simulink model "Doppelpendel_EKF"  (R2020b)
settings: Solver=ode45  StartTime=0.0  StopTime=10  EnableMultiTasking=on
undefined symbols (not defined in the file or in its folder): parDP, parEKF, parLQR
libraries: cstblocks x3
(part 2 of 2)

== matlab function Doppelpendel_EKF/Regler/LQR+EKF ==
  settings: updateMethod=DISCRETE  sampleTime=parLQR.Ta
  data: Switch_Rueckfuehrung input; statesd input; states input; uFF input; uG output; parDP parameter; parLQR parameter; parEKF parameter; xestout output; e_phi1 output; e_s output; e output; Pplus output
function [uG,xestout,e_phi1,e_s,e,Pplus]  = LQG(Switch_Rueckfuehrung,statesd,states,uFF,parDP,parLQR,parEKF)

%Anfangsbedinungen = Ruhelagen
persistent xI
if isempty(xI) xI = double(0); end

persistent xminus
if isempty(xminus)xminus = [parEKF.phi10;parEKF.omega10;parEKF.phi20;parEKF.omega20;parEKF.s0;parEKF.w0]; end

persistent Pminus
if isempty( Pminus) Pminus = diag([parEKF.delta,parEKF.delta,parEKF.delta,parEKF.delta,parEKF.delta,parEKF.delta]); end

%Ausgang
xestout=xminus;

%%%%%%%%%%%%%%%%%%%%%%%%%%%%%%%%%%%%%%%%%%%%%%%%%%%%%%%%%%%%%%%%%%%%%%%%%%%
%LQR-Regler
%%%%%%%%%%%%%%%%%%%%%%%%%%%%%%%%%%%%%%%%%%%%%%%%%%%%%%%%%%%%%%%%%%%%%%%%%%%

% Folgendes hier bitte ausführen:
% 1.) PI-Zustandsregler einfügen
    xI = xI + (statesd(5) - xestout(5));
    %Gesamtrückführung
    uFB = parLQR.kx*(xestout - statesd) + parLQR.kI * xI;
    uG = uFB + uFF;  

%%%%%%%%%%%%%%%%%%%%%%%%%%%%%%%%%%%%%%%%%%%%%%%%%%%%%%%%%%%%%%%%%%%%%%%%%%%
%EKF
%%%%%%%%%%%%%%%%%%%%%%%%%%%%%%%%%%%%%%%%%%%%%%%%%%%%%%%%%%%%%%%%%%%%%%%%%%%

% Folgendes hier bitte ausführen:
% 1.) Extended-Kalman-Filter einfügen
    C_k = [1 0 0 0 0 0; 0 0 0 0 1 0];
    % Hk = 0;
    %Korrekturschritt
    L_k = Pminus*C_k' / (C_k*Pminus*C_k' + parEKF.Rn);
    xplus = xminus + L_k*( [states(1); states(5)] - [ xestout(1); xestout(5)] );
    Pplus = (eye(6) - L_k*C_k) * Pminus;

    %Prädiktorschritt
    Phi_k = eye(6) + parDP.Ta*fcnAsys(xplus,uG,parDP);
    xminus = xplus + parDP.Ta*fcnfx(xplus,uG,parDP);
    Pminus = Phi_k*Pplus*Phi_k' + parEKF.Qn;


    e_phi1 = states(1) - xminus(1);
    e_s = states(5)- xminus(5);
    e = [e_phi1 ;0; 0; 0; e_s ;0];

end

%% Rechte Seite
function fx = fcnfx(xplus,uG,parDP)

    InvD11 = parDP.m2*parDP.a2*parDP.a2+parDP.J2;
    InvD12 = -parDP.m2*parDP.l1*parDP.a2*cos(xplus(1)-xplus(3));
    InvD22 = parDP.J1+parDP.a1*parDP.a1*parDP.m1+parDP.m2*parDP.l1*parDP.l1;
    den    = (parDP.J1+parDP.a1*parDP.a1*parDP.m1+parDP.m2*parDP.l1*parDP.l1)*(parDP.m2*parDP.a2*parDP.a2+parDP.J2)-parDP.m2*parDP.m2*parDP.l1*parDP.l1*parDP.a2*parDP.a2*(cos(xplus(1)-xplus(3)))^2;
    gg1    = parDP.d2*xplus(2)-parDP.d2*xplus(4)-parDP.m2*parDP.l1*cos(xplus(1))*uG-parDP.m1*parDP.g*parDP.a1*sin(xplus(1))-parDP.m2*parDP.g*parDP.l1*sin(xplus(1))-parDP.m1*parDP.a1*cos(xplus(1))*uG+parDP.d1*xplus(2)+parDP.m2*parDP.l1*parDP.a2*xplus(4)*xplus(4)*sin(xplus(1)-xplus(3));
    gg2    = -parDP.m2*parDP.g*parDP.a2*sin(xplus(3))-parDP.m2*parDP.a2*cos(xplus(3))*uG-parDP.m2*parDP.a2*parDP.l1*xplus(2)*xplus(2)*sin(xplus(1)-xplus(3))+parDP.d2*xplus(4)-parDP.d2*xplus(2);

        fx = [xplus(2);
              -1/den*(InvD11*gg1+InvD12*gg2);
              xplus(4);
              -1/den*(InvD12*gg1+InvD22*gg2);
              xplus(6);
              uG];
              
end
%% linearisierte Systemmatrix

function Asyslin = fcnAsys(xplus,u,parDP) %% linearisierte Systemmatrix

    Asyslin = [0 1 0 0 0 0;
               -0.1e1 / (parDP.J1 * parDP.m2 * parDP.a2 ^ 2 + parDP.J1 * parDP.J2 + parDP.a1 ^ 2 * parDP.m1 * parDP.m2 * parDP.a2 ^ 2 + parDP.a1 ^ 2 * parDP.m1 * parDP.J2 + parDP.m2 ^ 2 * parDP.l1 ^ 2 * parDP.a2 ^ 2 + parDP.m2 * parDP.l1 ^ 2 * parDP.J2 - parDP.m2 ^ 2 * parDP.l1 ^ 2 * parDP.a2 ^ 2 * cos(xplus(1)) ^ 2 * cos(xplus(3)) ^ 2 - 0.2e1 * parDP.m2 ^ 2 * parDP.l1 ^ 2 * parDP.a2 ^ 2 * cos(xplus(1)) * cos(xplus(3)) * sin(xplus(1)) * sin(xplus(3)) - parDP.m2 ^ 2 * parDP.l1 ^ 2 * parDP.a2 ^ 2 * sin(xplus(1)) ^ 2 * sin(xplus(3)) ^ 2) ^ 2 * (-parDP.d2 * xplus(2) * parDP.m2 * parDP.a2 ^ 2 + parDP.d2 * xplus(4) * parDP.m2 * parDP.a2 ^ 2 - parDP.d1 * xplus(2) * parDP.m2 * parDP.a2 ^ 2 + parDP.m2 ^ 2 * parDP.a2 ^ 3 * sin(xplus(3)) * xplus(4) * parDP.l1 * cos(xplus(1)) * xplus(2) - parDP.m2 ^ 2 * parDP.a2 ^ 3 * cos(xplus(3)) * xplus(4) * parDP.l1 * sin(xplus(1)) * xplus(2) + parDP.m1 * parDP.a1 * sin(xplus(1)) * xplus(2) * xplus(6) * parDP.m2 * parDP.a2 ^ 2 - parDP.m2 ^ 2 * parDP.l1 * parDP.a2 ^ 2 * cos(xplus(1)) * cos(xplus(3)) * parDP.g * sin(xplus(3)) - parDP.m2 ^ 2 * parDP.l1 * parDP.a2 ^ 2 * sin(xplus(1)) * sin(xplus(3)) ^ 2 * xplus(4) * xplus(6) - parDP.m2 ^ 2 * parDP.l1 * parDP.a2 ^ 2 * sin(xplus(1)) * sin(xplus(3)) * cos(xplus(3)) * u + parDP.m2 * parDP.l1 * parDP.a2 * cos(xplus(1)) * cos(xplus(3)) * parDP.d2 * xplus(4) - parDP.m2 * parDP.l1 * parDP.a2 * cos(xplus(1)) * cos(xplus(3)) * parDP.d2 * xplus(2) + parDP.m2 * parDP.l1 * parDP.a2 * sin(xplus(1)) * sin(xplus(3)) * parDP.d2 * xplus(4) - parDP.m2 * parDP.l1 * parDP.a2 * sin(xplus(1)) * sin(xplus(3)) * parDP.d2 * xplus(2) + parDP.m2 ^ 2 * parDP.l1 * cos(xplus(1)) * u * parDP.a2 ^ 2 + parDP.m2 * parDP.l1 * cos(xplus(1)) * u * parDP.J2 + parDP.m1 * parDP.g * parDP.a1 * sin(xplus(1)) * parDP.J2 + parDP.m2 ^ 2 * parDP.g * parDP.l1 * sin(xplus(1)) * parDP.a2 ^ 2 + parDP.m2 * parDP.g * parDP.l1 * sin(xplus(1)) * parDP.J2 + parDP.m1 * parDP.a1 * cos(xplus(1)) * u * parDP.J2 + parDP.m1 * parDP.g * parDP.a1 * sin(xplus(1)) * parDP.m2 * parDP.a2 ^ 2 + parDP.m1 * parDP.a1 * cos(xplus(1)) * u * parDP.m2 * parDP.a2 ^ 2 + parDP.m1 * parDP.a1 * sin(xplus(1)) * xplus(2) * xplus(6) * parDP.J2 + parDP.m2 ^ 2 * parDP.l1 * sin(xplus(1)) * xplus(2) * xplus(6) * parDP.a2 ^ 2 + parDP.m2 * parDP.l1 * sin(xplus(1)) * xplus(2) * xplus(6) * parDP.J2 - parDP.m2 ^ 2 * parDP.l1 * parDP.a2 ^ 2 * cos(xplus(1)) * cos(xplus(3)) ^ 2 * u - parDP.m2 ^ 2 * parDP.l1 * parDP.a2 ^ 2 * sin(xplus(1)) * sin(xplus(3)) ^ 2 * parDP.g - parDP.d2 * xplus(2) * parDP.J2 - parDP.d1 * xplus(2) * parDP.J2 + parDP.d2 * xplus(4) * parDP.J2 + parDP.m2 ^ 2 * parDP.l1 ^ 2 * parDP.a2 ^ 2 * cos(xplus(1)) ^ 2 * cos(xplus(3)) * sin(xplus(3)) * xplus(4) * xplus(2) + parDP.m2 ^ 2 * parDP.l1 ^ 2 * parDP.a2 ^ 2 * sin(xplus(1)) * sin(xplus(3)) ^ 2 * xplus(4) * cos(xplus(1)) * xplus(2) - parDP.m2 ^ 2 * parDP.l1 ^ 2 * parDP.a2 ^ 2 * sin(xplus(1)) ^ 2 * sin(xplus(3)) * cos(xplus(3)) * xplus(4) * xplus(2) - parDP.m2 ^ 2 * parDP.l1 ^ 2 * parDP.a2 ^ 2 * cos(xplus(1)) * cos(xplus(3)) ^ 2 * xplus(4) * sin(xplus(1)) * xplus(2) + parDP.m2 * parDP.a2 * sin(xplus(3)) * xplus(4) * parDP.l1 * cos(xplus(1)) * xplus(2) * parDP.J2 - parDP.m2 * parDP.a2 * cos(xplus(3)) * xplus(4) * parDP.l1 * sin(xplus(1)) * xplus(2) * parDP.J2 - parDP.m2 ^ 2 * parDP.l1 * parDP.a2 ^ 2 * cos(xplus(1)) * cos(xplus(3)) * sin(xplus(3)) * xplus(4) * xplus(6)) * (0.2e1 * parDP.m2 ^ 2 * parDP.l1 ^ 2 * parDP.a2 ^ 2 * cos(xplus(1)) * cos(xplus(3)) ^ 2 * sin(xplus(1)) + 0.2e1 * parDP.m2 ^ 2 * parDP.l1 ^ 2 * parDP.a2 ^ 2 * sin(xplus(1)) ^ 2 * cos(xplus(3)) * sin(xplus(3)) - 0.2e1 * parDP.m2 ^ 2 * parDP.l1 ^ 2 * parDP.a2 ^ 2 * cos(xplus(1)) ^ 2 * cos(xplus(3)) * sin(xplus(3)) - 0.2e1 * parDP.m2 ^ 2 * parDP.l1 ^ 2 * parDP.a2 ^ 2 * sin(xplus(1)) * sin(xplus(3)) ^ 2 * cos(xplus(1))) + 0.1e1 / (parDP.J1 * parDP.m2 * parDP.a2 ^ 2 + parDP.J1 * parDP.J2 + parDP.a1 ^ 2 * parDP.m1 * parDP.m2 * parDP.a2 ^ 2 + parDP.a1 ^ 2 * parDP.m1 * parDP.J2 + parDP.m2 ^ 2 * parDP.l1 ^ 2 * parDP.a2 ^ 2 + parDP.m2 * parDP.l1 ^ 2 * parDP.J2 - parDP.m2 ^ 2 * parDP.l1 ^ 2 * parDP.a2 ^ 2 * cos(xplus(1)) ^ 2 * cos(xplus(3)) ^ 2 - 0.2e1 * parDP.m2 ^ 2 * parDP.l1 ^ 2 * parDP.a2 ^ 2 * cos(xplus(1)) * cos(xplus(3)) * sin(xplus(1)) * sin(xplus(3)) - parDP.m2 ^ 2 * parDP.l1 ^ 2 * parDP.a2 ^ 2 * sin(xplus(1)) ^ 2 * sin(xplus(3)) ^ 2) * (-parDP.m2 ^ 2 * parDP.a2 ^ 3 * sin(xplus(3)) * xplus(4) * parDP.l1 * sin(xplus(1)) * xplus(2) - parDP.m2 ^ 2 * parDP.a2 ^ 3 * cos(xplus(3)) * xplus(4) * parDP.l1 * cos(xplus(1)) * xplus(2) + parDP.m1 * parDP.a1 * cos(xplus(1)) * xplus(2) * xplus(6) * parDP.m2 * parDP.a2 ^ 2 + parDP.m2 ^ 2 * parDP.l1 * parDP.a2 ^ 2 * sin(xplus(1)) * cos(xplus(3)) * parDP.g * sin(xplus(3)) - parDP.m2 ^ 2 * parDP.l1 * parDP.a2 ^ 2 * cos(xplus(1)) * sin(xplus(3)) ^ 2 * xplus(4) * xplus(6) - parDP.m2 ^ 2 * parDP.l1 * sin(xplus(1)) * u * parDP.a2 ^ 2 - parDP.m2 ^ 2 * parDP.l1 * parDP.a2 ^ 2 * cos(xplus(1)) * sin(xplus(3)) * cos(xplus(3)) * u - parDP.m2 * parDP.l1 * parDP.a2 * sin(xplus(1)) * cos(xplus(3)) * parDP.d2 * xplus(4) + parDP.m2 * parDP.l1 * parDP.a2 * sin(xplus(1)) * cos(xplus(3)) * parDP.d2 * xplus(2) + parDP.m2 * parDP.l1 * parDP.a2 * cos(xplus(1)) * sin(xplus(3)) * parDP.d2 * xplus(4) - parDP.m2 * parDP.l1 * parDP.a2 * cos(xplus(1)) * sin(xplus(3)) * parDP.d2 * xplus(2) - parDP.m2 ^ 2 * parDP.l1 ^ 2 * parDP.a2 ^ 2 * sin(xplus(1)) ^ 2 * sin(xplus(3)) ^ 2 * xplus(4) * xplus(2) + parDP.m2 ^ 2 * parDP.l1 ^ 2 * parDP.a2 ^ 2 * sin(xplus(1)) ^ 2 * cos(xplus(3)) ^ 2 * xplus(4) * xplus(2) + parDP.m1 * parDP.g * parDP.a1 * cos(xplus(1)) * parDP.m2 * parDP.a2 ^ 2 - parDP.m1 * parDP.a1 * sin(xplus(1)) * u * parDP.m2 * parDP.a2 ^ 2 + parDP.m1 * parDP.a1 * cos(xplus(1)) * xplus(2) * xplus(6) * parDP.J2 + parDP.m2 ^ 2 * parDP.l1 * cos(xplus(1)) * xplus(2) * xplus(6) * parDP.a2 ^ 2 + parDP.m2 * parDP.l1 * cos(xplus(1)) * xplus(2) * xplus(6) * parDP.J2 + parDP.m2 ^ 2 * parDP.l1 * parDP.a2 ^ 2 * sin(xplus(1)) * cos(xplus(3)) ^ 2 * u - parDP.m2 ^ 2 * parDP.l1 * parDP.a2 ^ 2 * cos(xplus(1)) * sin(xplus(3)) ^ 2 * parDP.g - parDP.m2 * parDP.l1 * sin(xplus(1)) * u * parDP.J2 + parDP.m1 * parDP.g * parDP.a1 * cos(xplus(1)) * parDP.J2 + parDP.m2 ^ 2 * parDP.g * parDP.l1 * cos(xplus(1)) * parDP.a2 ^ 2 + parDP.m2 * parDP.g * parDP.l1 * cos(xplus(1)) * parDP.J2 - parDP.m1 * parDP.a1 * sin(xplus(1)) * u * parDP.J2 - 0.4e1 * parDP.m2 ^ 2 * parDP.l1 ^ 2 * parDP.a2 ^ 2 * cos(xplus(1)) * cos(xplus(3)) * sin(xplus(3)) * xplus(4) * xplus(2) * sin(xplus(1)) + parDP.m2 ^ 2 * parDP.l1 ^ 2 * parDP.a2 ^ 2 * cos(xplus(1)) ^ 2 * sin(xplus(3)) ^ 2 * xplus(4) * xplus(2) - parDP.m2 ^ 2 * parDP.l1 ^ 2 * parDP.a2 ^ 2 * cos(xplus(1)) ^ 2 * cos(xplus(3)) ^ 2 * xplus(4) * xplus(2) - parDP.m2 * parDP.a2 * sin(xplus(3)) * xplus(4) * parDP.l1 * sin(xplus(1)) * xplus(2) * parDP.J2 - parDP.m2 * parDP.a2 * cos(xplus(3)) * xplus(4) * parDP.l1 * cos(xplus(1)) * xplus(2) * parDP.J2 + parDP.m2 ^ 2 * parDP.l1 * parDP.a2 ^ 2 * sin(xplus(1)) * cos(xplus(3)) * sin(xplus(3)) * xplus(4) * xplus(6)) 0.1e1 / (parDP.J1 * parDP.m2 * parDP.a2 ^ 2 + parDP.J1 * parDP.J2 + parDP.a1 ^ 2 * parDP.m1 * parDP.m2 * parDP.a2 ^ 2 + parDP.a1 ^ 2 * parDP.m1 * parDP.J2 + parDP.m2 ^ 2 * parDP.l1 ^ 2 * parDP.a2 ^ 2 + parDP.m2 * parDP.l1 ^ 2 * parDP.J2 - parDP.m2 ^ 2 * parDP.l1 ^ 2 * parDP.a2 ^ 2 * cos(xplus(1)) ^ 2 * cos(xplus(3)) ^ 2 - 0.2e1 * parDP.m2 ^ 2 * parDP.l1 ^ 2 * parDP.a2 ^ 2 * cos(xplus(1)) * cos(xplus(3)) * sin(xplus(1)) * sin(xplus(3)) - parDP.m2 ^ 2 * parDP.l1 ^ 2 * parDP.a2 ^ 2 * sin(xplus(1)) ^ 2 * sin(xplus(3)) ^ 2) * (-parDP.d2 * parDP.m2 * parDP.a2 ^ 2 - parDP.d1 * parDP.m2 * parDP.a2 ^ 2 + parDP.m2 ^ 2 * parDP.a2 ^ 3 * sin(xplus(3)) * xplus(4) * parDP.l1 * cos(xplus(1)) - parDP.m2 ^ 2 * parDP.a2 ^ 3 * cos(xplus(3)) * xplus(4) * parDP.l1 * sin(xplus(1)) + parDP.m1 * parDP.a1 * sin(xplus(1)) * xplus(6) * parDP.m2 * parDP.a2 ^ 2 - parDP.m2 * parDP.l1 * parDP.a2 * cos(xplus(1)) * cos(xplus(3)) * parDP.d2 - parDP.m2 * parDP.l1 * parDP.a2 * sin(xplus(1)) * sin(xplus(3)) * parDP.d2 + parDP.m1 * parDP.a1 * sin(xplus(1)) * xplus(6) * parDP.J2 + parDP.m2 ^ 2 * parDP.l1 * sin(xplus(1)) * xplus(6) * parDP.a2 ^ 2 + parDP.m2 * parDP.l1 * sin(xplus(1)) * xplus(6) * parDP.J2 - parDP.d2 * parDP.J2 - parDP.d1 * parDP.J2 + parDP.m2 ^ 2 * parDP.l1 ^ 2 * parDP.a2 ^ 2 * cos(xplus(1)) ^ 2 * cos(xplus(3)) * sin(xplus(3)) * xplus(4) + parDP.m2 ^ 2 * parDP.l1 ^ 2 * parDP.a2 ^ 2 * sin(xplus(1)) * sin(xplus(3)) ^ 2 * xplus(4) * cos(xplus(1)) - parDP.m2 ^ 2 * parDP.l1 ^ 2 * parDP.a2 ^ 2 * sin(xplus(1)) ^ 2 * sin(xplus(3)) * cos(xplus(3)) * xplus(4) - parDP.m2 ^ 2 * parDP.l1 ^ 2 * parDP.a2 ^ 2 * cos(xplus(1)) * cos(xplus(3)) ^ 2 * xplus(4) * sin(xplus(1)) + parDP.m2 * parDP.a2 * sin(xplus(3)) * xplus(4) * parDP.l1 * cos(xplus(1)) * parDP.J2 - parDP.m2 * parDP.a2 * cos(xplus(3)) * xplus(4) * parDP.l1 * sin(xplus(1)) * parDP.J2) -0.1e1 / (parDP.J1 * parDP.m2 * parDP.a2 ^ 2 + parDP.J1 * parDP.J2 + parDP.a1 ^ 2 * parDP.m1 * parDP.m2 * parDP.a2 ^ 2 + parDP.a1 ^ 2 * parDP.m1 * parDP.J2 + parDP.m2 ^ 2 * parDP.l1 ^ 2 * parDP.a2 ^ 2 + parDP.m2 * parDP.l1 ^ 2 * parDP.J2 - parDP.m2 ^ 2 * parDP.l1 ^ 2 * parDP.a2 ^ 2 * cos(xplus(1)) ^ 2 * cos(xplus(3)) ^ 2 - 0.2e1 * parDP.m2 ^ 2 * parDP.l1 ^ 2 * parDP.a2 ^ 2 * cos(xplus(1)) * cos(xplus(3)) * sin(xplus(1)) * sin(xplus(3)) - parDP.m2 ^ 2 * parDP.l1 ^ 2 * parDP.a2 ^ 2 * sin(xplus(1)) ^ 2 * sin(xplus(3)) ^ 2) ^ 2 * (-parDP.d2 * xplus(2) * parDP.m2 * parDP.a2 ^ 2 + parDP.d2 * xplus(4) * parDP.m2 * parDP.a2 ^ 2 - parDP.d1 * xplus(2) * parDP.m2 * parDP.a2 ^ 2 + parDP.m2 ^ 2 * parDP.a2 ^ 3 * sin(xplus(3)) * xplus(4) * parDP.l1 * cos(xplus(1)) * xplus(2) - parDP.m2 ^ 2 * parDP.a2 ^ 3 * cos(xplus(3)) * xplus(4) * parDP.l1 * sin(xplus(1)) * xplus(2) + parDP.m1 * parDP.a1 * sin(xplus(1)) * xplus(2) * xplus(6) * parDP.m2 * parDP.a2 ^ 2 - parDP.m2 ^ 2 * parDP.l1 * parDP.a2 ^ 2 * cos(xplus(1)) * cos(xplus(3)) * parDP.g * sin(xplus(3)) - parDP.m2 ^ 2 * parDP.l1 * parDP.a2 ^ 2 * sin(xplus(1)) * sin(xplus(3)) ^ 2 * xplus(4) * xplus(6) - parDP.m2 ^ 2 * parDP.l1 * parDP.a2 ^ 2 * sin(xplus(1)) * sin(xplus(3)) * cos(xplus(3)) * u + parDP.m2 * parDP.l1 * parDP.a2 * cos(xplus(1)) * cos(xplus(3)) * parDP.d2 * xplus(4) - parDP.m2 * parDP.l1 * parDP.a2 * cos(xplus(1)) * cos(xplus(3)) * parDP.d2 * xplus(2) + parDP.m2 * parDP.l1 * parDP.a2 * sin(xplus(1)) * sin(xplus(3)) * parDP.d2 * xplus(4) - parDP.m2 * parDP.l1 * parDP.a2 * sin(xplus(1)) * sin(xplus(3)) * parDP.d2 * xplus(2) + parDP.m2 ^ 2 * parDP.l1 * cos(xplus(1)) * u * parDP.a2 ^ 2 + parDP.m2 * parDP.l1 * cos(xplus(1)) * u * parDP.J2 + parDP.m1 * parDP.g * parDP.a1 * sin(xplus(1)) * parDP.J2 + parDP.m2 ^ 2 * parDP.g * parDP.l1 * sin(xplus(1)) * parDP.a2 ^ 2 + parDP.m2 * parDP.g * parDP.l1 * sin(xplus(1)) * parDP.J2 + parDP.m1 * parDP.a1 * cos(xplus(1)) * u * parDP.J2 + parDP.m1 * parDP.g * parDP.a1 * sin(xplus(1)) * parDP.m2 * parDP.a2 ^ 2 + parDP.m1 * parDP.a1 * cos(xplus(1)) * u * parDP.m2 * parDP.a2 ^ 2 + parDP.m1 * parDP.a1 * sin(xplus(1)) * xplus(2) * xplus(6) * parDP.J2 + parDP.m2 ^ 2 * parDP.l1 * sin(xplus(1)) * xplus(2) * xplus(6) * parDP.a2 ^ 2 + parDP.m2 * parDP.l1 * sin(xplus(1)) * xplus(2) * xplus(6) * parDP.J2 - parDP.m2 ^ 2 * parDP.l1 * parDP.a2 ^ 2 * cos(xplus(1)) * cos(xplus(3)) ^ 2 * u - parDP.m2 ^ 2 * parDP.l1 * parDP.a2 ^ 2 * sin(xplus(1)) * sin(xplus(3)) ^ 2 * parDP.g - parDP.d2 * xplus(2) * parDP.J2 - parDP.d1 * xplus(2) * parDP.J2 + parDP.d2 * xplus(4) * parDP.J2 + parDP.m2 ^ 2 * parDP.l1 ^ 2 * parDP.a2 ^ 2 * cos(xplus(1)) ^ 2 * cos(xplus(3)) * sin(xplus(3)) * xplus(4) * xplus(2) + parDP.m2 ^ 2 * parDP.l1 ^ 2 * parDP.a2 ^ 2 * sin(xplus(1)) * sin(xplus(3)) ^ 2 * xplus(4) * cos(xplus(1)) * xplus(2) - parDP.m2 ^ 2 * parDP.l1 ^ 2 * parDP.a2 ^ 2 * sin(xplus(1)) ^ 2 * sin(xplus(3)) * cos(xplus(3)) * xplus(4) * xplus(2) - parDP.m2 ^ 2 * parDP.l1 ^ 2 * parDP.a2 ^ 2 * cos(xplus(1)) * cos(xplus(3)) ^ 2 * xplus(4) * sin(xplus(1)) * xplus(2) + parDP.m2 * parDP.a2 * sin(xplus(3)) * xplus(4) * parDP.l1 * cos(xplus(1)) * xplus(2) * parDP.J2 - parDP.m2 * parDP.a2 * cos(xplus(3)) * xplus(4) * parDP.l1 * sin(xplus(1)) * xplus(2) * parDP.J2 - parDP.m2 ^ 2 * parDP.l1 * parDP.a2 ^ 2 * cos(xplus(1)) * cos(xplus(3)) * sin(xplus(3)) * xplus(4) * xplus(6)) * (0.2e1 * parDP.m2 ^ 2 * parDP.l1 ^ 2 * parDP.a2 ^ 2 * cos(xplus(1)) ^ 2 * cos(xplus(3)) * sin(xplus(3)) + 0.2e1 * parDP.m2 ^ 2 * parDP.l1 ^ 2 * parDP.a2 ^ 2 * sin(xplus(1)) * sin(xplus(3)) ^ 2 * cos(xplus(1)) - 0.2e1 * parDP.m2 ^ 2 * parDP.l1 ^ 2 * parDP.a2 ^ 2 * cos(xplus(1)) * cos(xplus(3)) ^ 2 * sin(xplus(1)) - 0.2e1 * parDP.m2 ^ 2 * parDP.l1 ^ 2 * parDP.a2 ^ 2 * sin(xplus(1)) ^ 2 * cos(xplus(3)) * sin(xplus(3))) + 0.1e1 / (parDP.J1 * parDP.m2 * parDP.a2 ^ 2 + parDP.J1 * parDP.J2 + parDP.a1 ^ 2 * parDP.m1 * parDP.m2 * parDP.a2 ^ 2 + parDP.a1 ^ 2 * parDP.m1 * parDP.J2 + parDP.m2 ^ 2 * parDP.l1 ^ 2 * parDP.a2 ^ 2 + parDP.m2 * parDP.l1 ^ 2 * parDP.J2 - parDP.m2 ^ 2 * parDP.l1 ^ 2 * parDP.a2 ^ 2 * cos(xplus(1)) ^ 2 * cos(xplus(3)) ^ 2 - 0.2e1 * parDP.m2 ^ 2 * parDP.l1 ^ 2 * parDP.a2 ^ 2 * cos(xplus(1)) * cos(xplus(3)) * sin(xplus(1)) * sin(xplus(3)) - parDP.m2 ^ 2 * parDP.l1 ^ 2 * parDP.a2 ^ 2 * sin(xplus(1)) ^ 2 * sin(xplus(3)) ^ 2) * (parDP.m2 ^ 2 * parDP.a2 ^ 3 * cos(xplus(3)) * xplus(4) * parDP.l1 * cos(xplus(1)) * xplus(2) + parDP.m2 ^ 2 * parDP.a2 ^ 3 * sin(xplus(3)) * xplus(4) * parDP.l1 * sin(xplus(1)) * xplus(2) + parDP.m2 ^ 2 * parDP.l1 * parDP.a2 ^ 2 * cos(xplus(1)) * sin(xplus(3)) ^ 2 * parDP.g - parDP.m2 ^ 2 * parDP.l1 * parDP.a2 ^ 2 * cos(xplus(1)) * cos(xplus(3)) ^ 2 * parDP.g - 0.2e1 * parDP.m2 ^ 2 * parDP.l1 * parDP.a2 ^ 2 * sin(xplus(1)) * cos(xplus(3)) * sin(xplus(3)) * xplus(4) * xplus(6) - parDP.m2 ^ 2 * parDP.l1 * parDP.a2 ^ 2 * sin(xplus(1)) * cos(xplus(3)) ^ 2 * u + parDP.m2 ^ 2 * parDP.l1 * parDP.a2 ^ 2 * sin(xplus(1)) * sin(xplus(3)) ^ 2 * u - parDP.m2 * parDP.l1 * parDP.a2 * cos(xplus(1)) * sin(xplus(3)) * parDP.d2 * xplus(4) + parDP.m2 * parDP.l1 * parDP.a2 * cos(xplus(1)) * sin(xplus(3)) * parDP.d2 * xplus(2) + parDP.m2 * parDP.l1 * parDP.a2 * sin(xplus(1)) * cos(xplus(3)) * parDP.d2 * xplus(4) - parDP.m2 * parDP.l1 * parDP.a2 * sin(xplus(1)) * cos(xplus(3)) * parDP.d2 * xplus(2) + 0.2e1 * parDP.m2 ^ 2 * parDP.l1 * parDP.a2 ^ 2 * cos(xplus(1)) * sin(xplus(3)) * cos(xplus(3)) * u - 0.2e1 * parDP.m2 ^ 2 * parDP.l1 * parDP.a2 ^ 2 * sin(xplus(1)) * cos(xplus(3)) * parDP.g * sin(xplus(3)) - parDP.m2 ^ 2 * parDP.l1 ^ 2 * parDP.a2 ^ 2 * cos(xplus(1)) ^ 2 * sin(xplus(3)) ^ 2 * xplus(4) * xplus(2) + parDP.m2 ^ 2 * parDP.l1 ^ 2 * parDP.a2 ^ 2 * cos(xplus(1)) ^ 2 * cos(xplus(3)) ^ 2 * xplus(4) * xplus(2) + 0.4e1 * parDP.m2 ^ 2 * parDP.l1 ^ 2 * parDP.a2 ^ 2 * cos(xplus(1)) * cos(xplus(3)) * sin(xplus(3)) * xplus(4) * xplus(2) * sin(xplus(1)) - parDP.m2 ^ 2 * parDP.l1 ^ 2 * parDP.a2 ^ 2 * sin(xplus(1)) ^ 2 * cos(xplus(3)) ^ 2 * xplus(4) * xplus(2) + parDP.m2 ^ 2 * parDP.l1 ^ 2 * parDP.a2 ^ 2 * sin(xplus(1)) ^ 2 * sin(xplus(3)) ^ 2 * xplus(4) * xplus(2) + parDP.m2 * parDP.a2 * cos(xplus(3)) * xplus(4) * parDP.l1 * cos(xplus(1)) * xplus(2) * parDP.J2 + parDP.m2 * parDP.a2 * sin(xplus(3)) * xplus(4) * parDP.l1 * sin(xplus(1)) * xplus(2) * parDP.J2 + parDP.m2 ^ 2 * parDP.l1 * parDP.a2 ^ 2 * cos(xplus(1)) * sin(xplus(3)) ^ 2 * xplus(4) * xplus(6) - parDP.m2 ^ 2 * parDP.l1 * parDP.a2 ^ 2 * cos(xplus(1)) * cos(xplus(3)) ^ 2 * xplus(4) * xplus(6)) 0.1e1 / (parDP.J1 * parDP.m2 * parDP.a2 ^ 2 + parDP.J1 * parDP.J2 + parDP.a1 ^ 2 * parDP.m1 * parDP.m2 * parDP.a2 ^ 2 + parDP.a1 ^ 2 * parDP.m1 * parDP.J2 + parDP.m2 ^ 2 * parDP.l1 ^ 2 * parDP.a2 ^ 2 + parDP.m2 * parDP.l1 ^ 2 * parDP.J2 - parDP.m2 ^ 2 * parDP.l1 ^ 2 * parDP.a2 ^ 2 * cos(xplus(1)) ^ 2 * cos(xplus(3)) ^ 2 - 0.2e1 * parDP.m2 ^ 2 * parDP.l1 ^ 2 * parDP.a2 ^ 2 * cos(xplus(1)) * cos(xplus(3)) * sin(xplus(1)) * sin(xplus(3)) - parDP.m2 ^ 2 * parDP.l1 ^ 2 * parDP.a2 ^ 2 * sin(xplus(1)) ^ 2 * sin(xplus(3)) ^ 2) * (parDP.d2 * parDP.m2 * parDP.a2 ^ 2 + parDP.m2 ^ 2 * parDP.a2 ^ 3 * sin(xplus(3)) * parDP.l1 * cos(xplus(1)) * xplus(2) - parDP.m2 ^ 2 * parDP.a2 ^ 3 * cos(xplus(3)) * parDP.l1 * sin(xplus(1)) * xplus(2) - parDP.m2 ^ 2 * parDP.l1 * parDP.a2 ^ 2 * sin(xplus(1)) * sin(xplus(3)) ^ 2 * xplus(6) + parDP.m2 * parDP.l1 * parDP.a2 * cos(xplus(1)) * cos(xplus(3)) * parDP.d2 + parDP.m2 * parDP.l1 * parDP.a2 * sin(xplus(1)) * sin(xplus(3)) * parDP.d2 + parDP.d2 * parDP.J2 + parDP.m2 ^ 2 * parDP.l1 ^ 2 * parDP.a2 ^ 2 * cos(xplus(1)) ^ 2 * cos(xplus(3)) * sin(xplus(3)) * xplus(2) + parDP.m2 ^ 2 * parDP.l1 ^ 2 * parDP.a2 ^ 2 * sin(xplus(1)) * sin(xplus(3)) ^ 2 * cos(xplus(1)) * xplus(2) - parDP.m2 ^ 2 * parDP.l1 ^ 2 * parDP.a2 ^ 2 * sin(xplus(1)) ^ 2 * sin(xplus(3)) * cos(xplus(3)) * xplus(2) - parDP.m2 ^ 2 * parDP.l1 ^ 2 * parDP.a2 ^ 2 * cos(xplus(1)) * cos(xplus(3)) ^ 2 * sin(xplus(1)) * xplus(2) + parDP.m2 * parDP.a2 * sin(xplus(3)) * parDP.l1 * cos(xplus(1)) * xplus(2) * parDP.J2 - parDP.m2 * parDP.a2 * cos(xplus(3)) * parDP.l1 * sin(xplus(1)) * xplus(2) * parDP.J2 - parDP.m2 ^ 2 * parDP.l1 * parDP.a2 ^ 2 * cos(xplus(1)) * cos(xplus(3)) * sin(xplus(3)) * xplus(6)) 0 0.1e1 / (parDP.J1 * parDP.m2 * parDP.a2 ^ 2 + parDP.J1 * parDP.J2 + parDP.a1 ^ 2 * parDP.m1 * parDP.m2 * parDP.a2 ^ 2 + parDP.a1 ^ 2 * parDP.m1 * parDP.J2 + parDP.m2 ^ 2 * parDP.l1 ^ 2 * parDP.a2 ^ 2 + parDP.m2 * parDP.l1 ^ 2 * parDP.J2 - parDP.m2 ^ 2 * parDP.l1 ^ 2 * parDP.a2 ^ 2 * cos(xplus(1)) ^ 2 * cos(xplus(3)) ^ 2 - 0.2e1 * parDP.m2 ^ 2 * parDP.l1 ^ 2 * parDP.a2 ^ 2 * cos(xplus(1)) * cos(xplus(3)) * sin(xplus(1)) * sin(xplus(3)) - parDP.m2 ^ 2 * parDP.l1 ^ 2 * parDP.a2 ^ 2 * sin(xplus(1)) ^ 2 * sin(xplus(3)) ^ 2) * (parDP.m1 * parDP.a1 * sin(xplus(1)) * xplus(2) * parDP.m2 * parDP.a2 ^ 2 - parDP.m2 ^ 2 * parDP.l1 * parDP.a2 ^ 2 * sin(xplus(1)) * sin(xplus(3)) ^ 2 * xplus(4) + parDP.m1 * parDP.a1 * sin(xplus(1)) * xplus(2) * parDP.J2 + parDP.m2 ^ 2 * parDP.l1 * sin(xplus(1)) * xplus(2) * parDP.a2 ^ 2 + parDP.m2 * parDP.l1 * sin(xplus(1)) * xplus(2) * parDP.J2 - parDP.m2 ^ 2 * parDP.l1 * parDP.a2 ^ 2 * cos(xplus(1)) * cos(xplus(3)) * sin(xplus(3)) * xplus(4))     ;
               0 0 0 1 0 0;
               (parDP.m2 * parDP.l1 * parDP.a2 * sin(xplus(1)) * cos(xplus(3)) * parDP.d2 * xplus(4) - parDP.m2 * parDP.l1 * parDP.a2 * sin(xplus(1)) * cos(xplus(3)) * parDP.d2 * xplus(2) - parDP.m2 * parDP.l1 * parDP.a2 * cos(xplus(1)) * sin(xplus(3)) * parDP.d2 * xplus(4) + parDP.m2 * parDP.l1 * parDP.a2 * cos(xplus(1)) * sin(xplus(3)) * parDP.d2 * xplus(2) + parDP.m2 ^ 2 * parDP.l1 ^ 2 * parDP.a2 ^ 2 * sin(xplus(1)) ^ 2 * sin(xplus(3)) ^ 2 * xplus(4) * xplus(2) - parDP.m2 ^ 2 * parDP.l1 ^ 2 * parDP.a2 ^ 2 * sin(xplus(1)) ^ 2 * cos(xplus(3)) ^ 2 * xplus(4) * xplus(2) + parDP.m2 ^ 2 * parDP.l1 ^ 2 * parDP.a2 * sin(xplus(1)) ^ 2 * sin(xplus(3)) * u + 0.4e1 * parDP.m2 ^ 2 * parDP.l1 ^ 2 * parDP.a2 ^ 2 * cos(xplus(1)) * cos(xplus(3)) * sin(xplus(3)) * xplus(4) * xplus(2) * sin(xplus(1)) - parDP.m2 ^ 2 * parDP.l1 ^ 2 * parDP.a2 ^ 2 * cos(xplus(1)) ^ 2 * sin(xplus(3)) ^ 2 * xplus(4) * xplus(2) + parDP.m2 ^ 2 * parDP.l1 ^ 2 * parDP.a2 ^ 2 * cos(xplus(1)) ^ 2 * cos(xplus(3)) ^ 2 * xplus(4) * xplus(2) + parDP.m2 ^ 2 * parDP.a2 * sin(xplus(3)) * xplus(4) * parDP.l1 ^ 3 * sin(xplus(1)) * xplus(2) - parDP.m2 * parDP.l1 * parDP.a2 * sin(xplus(1)) * cos(xplus(3)) * parDP.d1 * xplus(2) + parDP.m2 * parDP.l1 * parDP.a2 * cos(xplus(1)) * sin(xplus(3)) * parDP.d1 * xplus(2) - parDP.m2 ^ 2 * parDP.l1 ^ 2 * parDP.a2 * cos(xplus(1)) ^ 2 * cos(xplus(3)) * parDP.g - parDP.m2 ^ 2 * parDP.l1 ^ 2 * parDP.a2 * cos(xplus(1)) ^ 2 * sin(xplus(3)) * u + parDP.m2 ^ 2 * parDP.a2 * cos(xplus(3)) * xplus(4) * parDP.l1 ^ 3 * cos(xplus(1)) * xplus(2) - 0.2e1 * parDP.m2 ^ 2 * parDP.l1 ^ 2 * parDP.a2 * sin(xplus(1)) * sin(xplus(3)) * parDP.g * cos(xplus(1)) + 0.2e1 * parDP.m2 ^ 2 * parDP.l1 ^ 2 * parDP.a2 * cos(xplus(1)) * cos(xplus(3)) * u * sin(xplus(1)) + parDP.m2 ^ 2 * parDP.l1 ^ 2 * parDP.a2 * sin(xplus(1)) ^ 2 * cos(xplus(3)) * parDP.g - 0.2e1 * parDP.m2 ^ 2 * parDP.l1 ^ 2 * parDP.a2 * sin(xplus(1)) * sin(xplus(3)) * xplus(2) * xplus(6) * cos(xplus(1)) + 0.2e1 * parDP.m2 * parDP.l1 * parDP.a2 * cos(xplus(1)) * cos(xplus(3)) * parDP.m1 * parDP.a1 * u * sin(xplus(1)) + parDP.m2 ^ 2 * parDP.l1 ^ 2 * parDP.a2 * sin(xplus(1)) ^ 2 * cos(xplus(3)) * xplus(2) * xplus(6) - parDP.m2 * parDP.l1 * parDP.a2 * cos(xplus(1)) ^ 2 * cos(xplus(3)) * parDP.m1 * parDP.a1 * xplus(2) * xplus(6) + parDP.m2 * parDP.l1 * parDP.a2 * sin(xplus(1)) ^ 2 * cos(xplus(3)) * parDP.m1 * parDP.a1 * xplus(2) * xplus(6) - 0.2e1 * parDP.m2 * parDP.l1 * parDP.a2 * sin(xplus(1)) * sin(xplus(3)) * parDP.m1 * parDP.g * parDP.a1 * cos(xplus(1)) - parDP.m2 ^ 2 * parDP.l1 ^ 2 * parDP.a2 * cos(xplus(1)) ^ 2 * cos(xplus(3)) * xplus(2) * xplus(6) - parDP.m2 * parDP.l1 * parDP.a2 * cos(xplus(1)) ^ 2 * cos(xplus(3)) * parDP.m1 * parDP.g * parDP.a1 + parDP.m2 * parDP.l1 * parDP.a2 * sin(xplus(1)) ^ 2 * cos(xplus(3)) * parDP.m1 * parDP.g * parDP.a1 - parDP.m2 * parDP.l1 * parDP.a2 * cos(xplus(1)) ^ 2 * sin(xplus(3)) * parDP.m1 * parDP.a1 * u + parDP.m2 * parDP.l1 * parDP.a2 * sin(xplus(1)) ^ 2 * sin(xplus(3)) * parDP.m1 * parDP.a1 * u - 0.2e1 * parDP.m2 * parDP.l1 * parDP.a2 * sin(xplus(1)) * sin(xplus(3)) * parDP.m1 * parDP.a1 * xplus(2) * xplus(6) * cos(xplus(1)) + parDP.m2 * parDP.a2 * sin(xplus(3)) * xplus(4) * parDP.l1 * sin(xplus(1)) * xplus(2) * parDP.J1 + parDP.m2 * parDP.a2 * sin(xplus(3)) * xplus(4) * parDP.l1 * sin(xplus(1)) * xplus(2) * parDP.a1 ^ 2 * parDP.m1 + parDP.m2 * parDP.a2 * cos(xplus(3)) * xplus(4) * parDP.l1 * cos(xplus(1)) * xplus(2) * parDP.J1 + parDP.m2 * parDP.a2 * cos(xplus(3)) * xplus(4) * parDP.l1 * cos(xplus(1)) * xplus(2) * parDP.a1 ^ 2 * parDP.m1) / (parDP.J1 * parDP.m2 * parDP.a2 ^ 2 + parDP.J1 * parDP.J2 + parDP.a1 ^ 2 * parDP.m1 * parDP.m2 * parDP.a2 ^ 2 + parDP.a1 ^ 2 * parDP.m1 * parDP.J2 + parDP.m2 ^ 2 * parDP.l1 ^ 2 * parDP.a2 ^ 2 + parDP.m2 * parDP.l1 ^ 2 * parDP.J2 - parDP.m2 ^ 2 * parDP.l1 ^ 2 * parDP.a2 ^ 2 * cos(xplus(1)) ^ 2 * cos(xplus(3)) ^ 2 - 0.2e1 * parDP.m2 ^ 2 * parDP.l1 ^ 2 * parDP.a2 ^ 2 * cos(xplus(1)) * cos(xplus(3)) * sin(xplus(1)) * sin(xplus(3)) - parDP.m2 ^ 2 * parDP.l1 ^ 2 * parDP.a2 ^ 2 * sin(xplus(1)) ^ 2 * sin(xplus(3)) ^ 2) - (parDP.d2 * xplus(2) * parDP.m2 * parDP.l1 ^ 2 - parDP.d2 * xplus(4) * parDP.m2 * parDP.l1 ^ 2 - parDP.d2 * xplus(4) * parDP.a1 ^ 2 * parDP.m1 + parDP.d2 * xplus(2) * parDP.a1 ^ 2 * parDP.m1 - parDP.m2 ^ 2 * parDP.a2 * sin(xplus(3)) * xplus(4) * parDP.l1 ^ 3 * cos(xplus(1)) * xplus(2) - parDP.m2 * parDP.l1 * parDP.a2 * cos(xplus(1)) * cos(xplus(3)) * parDP.d2 * xplus(4) + parDP.m2 * parDP.l1 * parDP.a2 * cos(xplus(1)) * cos(xplus(3)) * parDP.d2 * xplus(2) - parDP.m2 * parDP.l1 * parDP.a2 * sin(xplus(1)) * sin(xplus(3)) * parDP.d2 * xplus(4) + parDP.m2 * parDP.l1 * parDP.a2 * sin(xplus(1)) * sin(xplus(3)) * parDP.d2 * xplus(2) + parDP.m2 * parDP.l1 * parDP.a2 * cos(xplus(1)) * cos(xplus(3)) * parDP.d1 * xplus(2) + parDP.m2 * parDP.l1 * parDP.a2 * sin(xplus(1)) * sin(xplus(3)) * parDP.d1 * xplus(2) - parDP.m2 ^ 2 * parDP.l1 ^ 2 * parDP.a2 * cos(xplus(1)) * cos(xplus(3)) * parDP.g * sin(xplus(1)) - parDP.m2 ^ 2 * parDP.l1 ^ 2 * parDP.a2 * sin(xplus(1)) * sin(xplus(3)) * cos(xplus(1)) * u + parDP.m2 ^ 2 * parDP.a2 * cos(xplus(3)) * xplus(4) * parDP.l1 ^ 3 * sin(xplus(1)) * xplus(2) - parDP.m2 ^ 2 * parDP.l1 ^ 2 * parDP.a2 * sin(xplus(1)) ^ 2 * sin(xplus(3)) * xplus(2) * xplus(6) + parDP.m2 * parDP.a2 * sin(xplus(3)) * xplus(4) * xplus(6) * parDP.a1 ^ 2 * parDP.m1 + parDP.m2 ^ 2 * parDP.g * parDP.a2 * sin(xplus(3)) * parDP.l1 ^ 2 + parDP.m2 * parDP.g * parDP.a2 * sin(xplus(3)) * parDP.J1 + parDP.m2 * parDP.a2 * cos(xplus(3)) * u * parDP.J1 + parDP.m2 ^ 2 * parDP.a2 * cos(xplus(3)) * u * parDP.l1 ^ 2 - parDP.m2 ^ 2 * parDP.l1 ^ 2 * parDP.a2 * sin(xplus(1)) ^ 2 * sin(xplus(3)) * parDP.g + parDP.m2 * parDP.a2 * sin(xplus(3)) * xplus(4) * xplus(6) * parDP.J1 + parDP.m2 ^ 2 * parDP.a2 * sin(xplus(3)) * xplus(4) * xplus(6) * parDP.l1 ^ 2 + parDP.m2 * parDP.g * parDP.a2 * sin(xplus(3)) * parDP.a1 ^ 2 * parDP.m1 + parDP.m2 * parDP.a2 * cos(xplus(3)) * u * parDP.a1 ^ 2 * parDP.m1 - parDP.m2 ^ 2 * parDP.l1 ^ 2 * parDP.a2 * cos(xplus(1)) ^ 2 * cos(xplus(3)) * u - parDP.d2 * xplus(4) * parDP.J1 + parDP.d2 * xplus(2) * parDP.J1 - parDP.m2 ^ 2 * parDP.l1 ^ 2 * parDP.a2 ^ 2 * cos(xplus(1)) ^ 2 * cos(xplus(3)) * sin(xplus(3)) * xplus(4) * xplus(2) - parDP.m2 ^ 2 * parDP.l1 ^ 2 * parDP.a2 ^ 2 * sin(xplus(1)) * sin(xplus(3)) ^ 2 * xplus(4) * cos(xplus(1)) * xplus(2) + parDP.m2 ^ 2 * parDP.l1 ^ 2 * parDP.a2 ^ 2 * sin(xplus(1)) ^ 2 * sin(xplus(3)) * cos(xplus(3)) * xplus(4) * xplus(2) + parDP.m2 ^ 2 * parDP.l1 ^ 2 * parDP.a2 ^ 2 * cos(xplus(1)) * cos(xplus(3)) ^ 2 * xplus(4) * sin(xplus(1)) * xplus(2) - parDP.m2 * parDP.l1 * parDP.a2 * cos(xplus(1)) ^ 2 * cos(xplus(3)) * parDP.m1 * parDP.a1 * u - parDP.m2 * parDP.l1 * parDP.a2 * cos(xplus(1)) * cos(xplus(3)) * parDP.m1 * parDP.a1 * sin(xplus(1)) * xplus(2) * xplus(6) - parDP.m2 * parDP.l1 * parDP.a2 * sin(xplus(1)) ^ 2 * sin(xplus(3)) * parDP.m1 * parDP.g * parDP.a1 - parDP.m2 ^ 2 * parDP.l1 ^ 2 * parDP.a2 * cos(xplus(1)) * cos(xplus(3)) * sin(xplus(1)) * xplus(2) * xplus(6) - parDP.m2 * parDP.l1 * parDP.a2 * cos(xplus(1)) * cos(xplus(3)) * parDP.m1 * parDP.g * parDP.a1 * sin(xplus(1)) - parDP.m2 * parDP.l1 * parDP.a2 * sin(xplus(1)) * sin(xplus(3)) * parDP.m1 * parDP.a1 * cos(xplus(1)) * u - parDP.m2 * parDP.l1 * parDP.a2 * sin(xplus(1)) ^ 2 * sin(xplus(3)) * parDP.m1 * parDP.a1 * xplus(2) * xplus(6) - parDP.m2 * parDP.a2 * sin(xplus(3)) * xplus(4) * parDP.l1 * cos(xplus(1)) * xplus(2) * parDP.J1 - parDP.m2 * parDP.a2 * sin(xplus(3)) * xplus(4) * parDP.l1 * cos(xplus(1)) * xplus(2) * parDP.a1 ^ 2 * parDP.m1 + parDP.m2 * parDP.a2 * cos(xplus(3)) * xplus(4) * parDP.l1 * sin(xplus(1)) * xplus(2) * parDP.J1 + parDP.m2 * parDP.a2 * cos(xplus(3)) * xplus(4) * parDP.l1 * sin(xplus(1)) * xplus(2) * parDP.a1 ^ 2 * parDP.m1) / (parDP.J1 * parDP.m2 * parDP.a2 ^ 2 + parDP.J1 * parDP.J2 + parDP.a1 ^ 2 * parDP.m1 * parDP.m2 * parDP.a2 ^ 2 + parDP.a1 ^ 2 * parDP.m1 * parDP.J2 + parDP.m2 ^ 2 * parDP.l1 ^ 2 * parDP.a2 ^ 2 + parDP.m2 * parDP.l1 ^ 2 * parDP.J2 - parDP.m2 ^ 2 * parDP.l1 ^ 2 * parDP.a2 ^ 2 * cos(xplus(1)) ^ 2 * cos(xplus(3)) ^ 2 - 0.2e1 * parDP.m2 ^ 2 * parDP.l1 ^ 2 * parDP.a2 ^ 2 * cos(xplus(1)) * cos(xplus(3)) * sin(xplus(1)) * sin(xplus(3)) - parDP.m2 ^ 2 * parDP.l1 ^ 2 * parDP.a2 ^ 2 * sin(xplus(1)) ^ 2 * sin(xplus(3)) ^ 2) ^ 2 * (0.2e1 * parDP.m2 ^ 2 * parDP.l1 ^ 2 * parDP.a2 ^ 2 * cos(xplus(1)) * cos(xplus(3)) ^ 2 * sin(xplus(1)) + 0.2e1 * parDP.m2 ^ 2 * parDP.l1 ^ 2 * parDP.a2 ^ 2 * sin(xplus(1)) ^ 2 * cos(xplus(3)) * sin(xplus(3)) - 0.2e1 * parDP.m2 ^ 2 * parDP.l1 ^ 2 * parDP.a2 ^ 2 * cos(xplus(1)) ^ 2 * cos(xplus(3)) * sin(xplus(3)) - 0.2e1 * parDP.m2 ^ 2 * parDP.l1 ^ 2 * parDP.a2 ^ 2 * sin(xplus(1)) * sin(xplus(3)) ^ 2 * cos(xplus(1))) (parDP.d2 * parDP.m2 * parDP.l1 ^ 2 + parDP.d2 * parDP.a1 ^ 2 * parDP.m1 - parDP.m2 ^ 2 * parDP.a2 * sin(xplus(3)) * xplus(4) * parDP.l1 ^ 3 * cos(xplus(1)) + parDP.m2 * parDP.l1 * parDP.a2 * cos(xplus(1)) * cos(xplus(3)) * parDP.d2 + parDP.m2 * parDP.l1 * parDP.a2 * sin(xplus(1)) * sin(xplus(3)) * parDP.d2 + parDP.m2 * parDP.l1 * parDP.a2 * cos(xplus(1)) * cos(xplus(3)) * parDP.d1 + parDP.m2 * parDP.l1 * parDP.a2 * sin(xplus(1)) * sin(xplus(3)) * parDP.d1 + parDP.m2 ^ 2 * parDP.a2 * cos(xplus(3)) * xplus(4) * parDP.l1 ^ 3 * sin(xplus(1)) - parDP.m2 ^ 2 * parDP.l1 ^ 2 * parDP.a2 * sin(xplus(1)) ^ 2 * sin(xplus(3)) * xplus(6) + parDP.d2 * parDP.J1 - parDP.m2 ^ 2 * parDP.l1 ^ 2 * parDP.a2 ^ 2 * cos(xplus(1)) ^ 2 * cos(xplus(3)) * sin(xplus(3)) * xplus(4) - parDP.m2 ^ 2 * parDP.l1 ^ 2 * parDP.a2 ^ 2 * sin(xplus(1)) * sin(xplus(3)) ^ 2 * xplus(4) * cos(xplus(1)) + parDP.m2 ^ 2 * parDP.l1 ^ 2 * parDP.a2 ^ 2 * sin(xplus(1)) ^ 2 * sin(xplus(3)) * cos(xplus(3)) * xplus(4) + parDP.m2 ^ 2 * parDP.l1 ^ 2 * parDP.a2 ^ 2 * cos(xplus(1)) * cos(xplus(3)) ^ 2 * xplus(4) * sin(xplus(1)) - parDP.m2 * parDP.l1 * parDP.a2 * cos(xplus(1)) * cos(xplus(3)) * parDP.m1 * parDP.a1 * sin(xplus(1)) * xplus(6) - parDP.m2 ^ 2 * parDP.l1 ^ 2 * parDP.a2 * cos(xplus(1)) * cos(xplus(3)) * sin(xplus(1)) * xplus(6) - parDP.m2 * parDP.l1 * parDP.a2 * sin(xplus(1)) ^ 2 * sin(xplus(3)) * parDP.m1 * parDP.a1 * xplus(6) - parDP.m2 * parDP.a2 * sin(xplus(3)) * xplus(4) * parDP.l1 * cos(xplus(1)) * parDP.J1 - parDP.m2 * parDP.a2 * sin(xplus(3)) * xplus(4) * parDP.l1 * cos(xplus(1)) * parDP.a1 ^ 2 * parDP.m1 + parDP.m2 * parDP.a2 * cos(xplus(3)) * xplus(4) * parDP.l1 * sin(xplus(1)) * parDP.J1 + parDP.m2 * parDP.a2 * cos(xplus(3)) * xplus(4) * parDP.l1 * sin(xplus(1)) * parDP.a1 ^ 2 * parDP.m1) / (parDP.J1 * parDP.m2 * parDP.a2 ^ 2 + parDP.J1 * parDP.J2 + parDP.a1 ^ 2 * parDP.m1 * parDP.m2 * parDP.a2 ^ 2 + parDP.a1 ^ 2 * parDP.m1 * parDP.J2 + parDP.m2 ^ 2 * parDP.l1 ^ 2 * parDP.a2 ^ 2 + parDP.m2 * parDP.l1 ^ 2 * parDP.J2 - parDP.m2 ^ 2 * parDP.l1 ^ 2 * parDP.a2 ^ 2 * cos(xplus(1)) ^ 2 * cos(xplus(3)) ^ 2 - 0.2e1 * parDP.m2 ^ 2 * parDP.l1 ^ 2 * parDP.a2 ^ 2 * cos(xplus(1)) * cos(xplus(3)) * sin(xplus(1)) * sin(xplus(3)) - parDP.m2 ^ 2 * parDP.l1 ^ 2 * parDP.a2 ^ 2 * sin(xplus(1)) ^ 2 * sin(xplus(3)) ^ 2) (-parDP.m2 * parDP.l1 * parDP.a2 * sin(xplus(1)) * cos(xplus(3)) * parDP.d2 * xplus(4) + parDP.m2 * parDP.l1 * parDP.a2 * sin(xplus(1)) * cos(xplus(3)) * parDP.d2 * xplus(2) + parDP.m2 * parDP.l1 * parDP.a2 * cos(xplus(1)) * sin(xplus(3)) * parDP.d2 * xplus(4) - parDP.m2 * parDP.l1 * parDP.a2 * cos(xplus(1)) * sin(xplus(3)) * parDP.d2 * xplus(2) - parDP.m2 ^ 2 * parDP.l1 ^ 2 * parDP.a2 ^ 2 * sin(xplus(1)) ^ 2 * sin(xplus(3)) ^ 2 * xplus(4) * xplus(2) + parDP.m2 ^ 2 * parDP.l1 ^ 2 * parDP.a2 ^ 2 * sin(xplus(1)) ^ 2 * cos(xplus(3)) ^ 2 * xplus(4) * xplus(2) - 0.4e1 * parDP.m2 ^ 2 * parDP.l1 ^ 2 * parDP.a2 ^ 2 * cos(xplus(1)) * cos(xplus(3)) * sin(xplus(3)) * xplus(4) * xplus(2) * sin(xplus(1)) + parDP.m2 ^ 2 * parDP.l1 ^ 2 * parDP.a2 ^ 2 * cos(xplus(1)) ^ 2 * sin(xplus(3)) ^ 2 * xplus(4) * xplus(2) - parDP.m2 ^ 2 * parDP.l1 ^ 2 * parDP.a2 ^ 2 * cos(xplus(1)) ^ 2 * cos(xplus(3)) ^ 2 * xplus(4) * xplus(2) - parDP.m2 ^ 2 * parDP.a2 * sin(xplus(3)) * u * parDP.l1 ^ 2 - parDP.m2 ^ 2 * parDP.a2 * sin(xplus(3)) * xplus(4) * parDP.l1 ^ 3 * sin(xplus(1)) * xplus(2) + parDP.m2 * parDP.l1 * parDP.a2 * sin(xplus(1)) * cos(xplus(3)) * parDP.d1 * xplus(2) - parDP.m2 * parDP.l1 * parDP.a2 * cos(xplus(1)) * sin(xplus(3)) * parDP.d1 * xplus(2) + parDP.m2 ^ 2 * parDP.l1 ^ 2 * parDP.a2 * cos(xplus(1)) ^ 2 * sin(xplus(3)) * u - parDP.m2 ^ 2 * parDP.a2 * cos(xplus(3)) * xplus(4) * parDP.l1 ^ 3 * cos(xplus(1)) * xplus(2) + parDP.m2 ^ 2 * parDP.l1 ^ 2 * parDP.a2 * sin(xplus(1)) * sin(xplus(3)) * parDP.g * cos(xplus(1)) - parDP.m2 ^ 2 * parDP.l1 ^ 2 * parDP.a2 * cos(xplus(1)) * cos(xplus(3)) * u * sin(xplus(1)) + parDP.m2 ^ 2 * parDP.g * parDP.a2 * cos(xplus(3)) * parDP.l1 ^ 2 + parDP.m2 * parDP.a2 * cos(xplus(3)) * xplus(4) * xplus(6) * parDP.a1 ^ 2 * parDP.m1 - parDP.m2 ^ 2 * parDP.l1 ^ 2 * parDP.a2 * sin(xplus(1)) ^ 2 * cos(xplus(3)) * parDP.g - parDP.m2 * parDP.a2 * sin(xplus(3)) * u * parDP.J1 + parDP.m2 * parDP.g * parDP.a2 * cos(xplus(3)) * parDP.J1 + parDP.m2 ^ 2 * parDP.l1 ^ 2 * parDP.a2 * sin(xplus(1)) * sin(xplus(3)) * xplus(2) * xplus(6) * cos(xplus(1)) + parDP.m2 * parDP.a2 * cos(xplus(3)) * xplus(4) * xplus(6) * parDP.J1 + parDP.m2 ^ 2 * parDP.a2 * cos(xplus(3)) * xplus(4) * xplus(6) * parDP.l1 ^ 2 + parDP.m2 * parDP.g * parDP.a2 * cos(xplus(3)) * parDP.a1 ^ 2 * parDP.m1 - parDP.m2 * parDP.a2 * sin(xplus(3)) * u * parDP.a1 ^ 2 * parDP.m1 - parDP.m2 * parDP.l1 * parDP.a2 * cos(xplus(1)) * cos(xplus(3)) * parDP.m1 * parDP.a1 * u * sin(xplus(1)) - parDP.m2 ^ 2 * parDP.l1 ^ 2 * parDP.a2 * sin(xplus(1)) ^ 2 * cos(xplus(3)) * xplus(2) * xplus(6) - parDP.m2 * parDP.l1 * parDP.a2 * sin(xplus(1)) ^ 2 * cos(xplus(3)) * parDP.m1 * parDP.a1 * xplus(2) * xplus(6) + parDP.m2 * parDP.l1 * parDP.a2 * sin(xplus(1)) * sin(xplus(3)) * parDP.m1 * parDP.g * parDP.a1 * cos(xplus(1)) - parDP.m2 * parDP.l1 * parDP.a2 * sin(xplus(1)) ^ 2 * cos(xplus(3)) * parDP.m1 * parDP.g * parDP.a1 + parDP.m2 * parDP.l1 * parDP.a2 * cos(xplus(1)) ^ 2 * sin(xplus(3)) * parDP.m1 * parDP.a1 * u + parDP.m2 * parDP.l1 * parDP.a2 * sin(xplus(1)) * sin(xplus(3)) * parDP.m1 * parDP.a1 * xplus(2) * xplus(6) * cos(xplus(1)) - parDP.m2 * parDP.a2 * sin(xplus(3)) * xplus(4) * parDP.l1 * sin(xplus(1)) * xplus(2) * parDP.J1 - parDP.m2 * parDP.a2 * sin(xplus(3)) * xplus(4) * parDP.l1 * sin(xplus(1)) * xplus(2) * parDP.a1 ^ 2 * parDP.m1 - parDP.m2 * parDP.a2 * cos(xplus(3)) * xplus(4) * parDP.l1 * cos(xplus(1)) * xplus(2) * parDP.J1 - parDP.m2 * parDP.a2 * cos(xplus(3)) * xplus(4) * parDP.l1 * cos(xplus(1)) * xplus(2) * parDP.a1 ^ 2 * parDP.m1) / (parDP.J1 * parDP.m2 * parDP.a2 ^ 2 + parDP.J1 * parDP.J2 + parDP.a1 ^ 2 * parDP.m1 * parDP.m2 * parDP.a2 ^ 2 + parDP.a1 ^ 2 * parDP.m1 * parDP.J2 + parDP.m2 ^ 2 * parDP.l1 ^ 2 * parDP.a2 ^ 2 + parDP.m2 * parDP.l1 ^ 2 * parDP.J2 - parDP.m2 ^ 2 * parDP.l1 ^ 2 * parDP.a2 ^ 2 * cos(xplus(1)) ^ 2 * cos(xplus(3)) ^ 2 - 0.2e1 * parDP.m2 ^ 2 * parDP.l1 ^ 2 * parDP.a2 ^ 2 * cos(xplus(1)) * cos(xplus(3)) * sin(xplus(1)) * sin(xplus(3)) - parDP.m2 ^ 2 * parDP.l1 ^ 2 * parDP.a2 ^ 2 * sin(xplus(1)) ^ 2 * sin(xplus(3)) ^ 2) - (parDP.d2 * xplus(2) * parDP.m2 * parDP.l1 ^ 2 - parDP.d2 * xplus(4) * parDP.m2 * parDP.l1 ^ 2 - parDP.d2 * xplus(4) * parDP.a1 ^ 2 * parDP.m1 + parDP.d2 * xplus(2) * parDP.a1 ^ 2 * parDP.m1 - parDP.m2 ^ 2 * parDP.a2 * sin(xplus(3)) * xplus(4) * parDP.l1 ^ 3 * cos(xplus(1)) * xplus(2) - parDP.m2 * parDP.l1 * parDP.a2 * cos(xplus(1)) * cos(xplus(3)) * parDP.d2 * xplus(4) + parDP.m2 * parDP.l1 * parDP.a2 * cos(xplus(1)) * cos(xplus(3)) * parDP.d2 * xplus(2) - parDP.m2 * parDP.l1 * parDP.a2 * sin(xplus(1)) * sin(xplus(3)) * parDP.d2 * xplus(4) + parDP.m2 * parDP.l1 * parDP.a2 * sin(xplus(1)) * sin(xplus(3)) * parDP.d2 * xplus(2) + parDP.m2 * parDP.l1 * parDP.a2 * cos(xplus(1)) * cos(xplus(3)) * parDP.d1 * xplus(2) + parDP.m2 * parDP.l1 * parDP.a2 * sin(xplus(1)) * sin(xplus(3)) * parDP.d1 * xplus(2) - parDP.m2 ^ 2 * parDP.l1 ^ 2 * parDP.a2 * cos(xplus(1)) * cos(xplus(3)) * parDP.g * sin(xplus(1)) - parDP.m2 ^ 2 * parDP.l1 ^ 2 * parDP.a2 * sin(xplus(1)) * sin(xplus(3)) * cos(xplus(1)) * u + parDP.m2 ^ 2 * parDP.a2 * cos(xplus(3)) * xplus(4) * parDP.l1 ^ 3 * sin(xplus(1)) * xplus(2) - parDP.m2 ^ 2 * parDP.l1 ^ 2 * parDP.a2 * sin(xplus(1)) ^ 2 * sin(xplus(3)) * xplus(2) * xplus(6) + parDP.m2 * parDP.a2 * sin(xplus(3)) * xplus(4) * xplus(6) * parDP.a1 ^ 2 * parDP.m1 + parDP.m2 ^ 2 * parDP.g * parDP.a2 * sin(xplus(3)) * parDP.l1 ^ 2 + parDP.m2 * parDP.g * parDP.a2 * sin(xplus(3)) * parDP.J1 + parDP.m2 * parDP.a2 * cos(xplus(3)) * u * parDP.J1 + parDP.m2 ^ 2 * parDP.a2 * cos(xplus(3)) * u * parDP.l1 ^ 2 - parDP.m2 ^ 2 * parDP.l1 ^ 2 * parDP.a2 * sin(xplus(1)) ^ 2 * sin(xplus(3)) * parDP.g + parDP.m2 * parDP.a2 * sin(xplus(3)) * xplus(4) * xplus(6) * parDP.J1 + parDP.m2 ^ 2 * parDP.a2 * sin(xplus(3)) * xplus(4) * xplus(6) * parDP.l1 ^ 2 + parDP.m2 * parDP.g * parDP.a2 * sin(xplus(3)) * parDP.a1 ^ 2 * parDP.m1 + parDP.m2 * parDP.a2 * cos(xplus(3)) * u * parDP.a1 ^ 2 * parDP.m1 - parDP.m2 ^ 2 * parDP.l1 ^ 2 * parDP.a2 * cos(xplus(1)) ^ 2 * cos(xplus(3)) * u - parDP.d2 * xplus(4) * parDP.J1 + parDP.d2 * xplus(2) * parDP.J1 - parDP.m2 ^ 2 * parDP.l1 ^ 2 * parDP.a2 ^ 2 * cos(xplus(1)) ^ 2 * cos(xplus(3)) * sin(xplus(3)) * xplus(4) * xplus(2) - parDP.m2 ^ 2 * parDP.l1 ^ 2 * parDP.a2 ^ 2 * sin(xplus(1)) * sin(xplus(3)) ^ 2 * xplus(4) * cos(xplus(1)) * xplus(2) + parDP.m2 ^ 2 * parDP.l1 ^ 2 * parDP.a2 ^ 2 * sin(xplus(1)) ^ 2 * sin(xplus(3)) * cos(xplus(3)) * xplus(4) * xplus(2) + parDP.m2 ^ 2 * parDP.l1 ^ 2 * parDP.a2 ^ 2 * cos(xplus(1)) * cos(xplus(3)) ^ 2 * xplus(4) * sin(xplus(1)) * xplus(2) - parDP.m2 * parDP.l1 * parDP.a2 * cos(xplus(1)) ^ 2 * cos(xplus(3)) * parDP.m1 * parDP.a1 * u - parDP.m2 * parDP.l1 * parDP.a2 * cos(xplus(1)) * cos(xplus(3)) * parDP.m1 * parDP.a1 * sin(xplus(1)) * xplus(2) * xplus(6) - parDP.m2 * parDP.l1 * parDP.a2 * sin(xplus(1)) ^ 2 * sin(xplus(3)) * parDP.m1 * parDP.g * parDP.a1 - parDP.m2 ^ 2 * parDP.l1 ^ 2 * parDP.a2 * cos(xplus(1)) * cos(xplus(3)) * sin(xplus(1)) * xplus(2) * xplus(6) - parDP.m2 * parDP.l1 * parDP.a2 * cos(xplus(1)) * cos(xplus(3)) * parDP.m1 * parDP.g * parDP.a1 * sin(xplus(1)) - parDP.m2 * parDP.l1 * parDP.a2 * sin(xplus(1)) * sin(xplus(3)) * parDP.m1 * parDP.a1 * cos(xplus(1)) * u - parDP.m2 * parDP.l1 * parDP.a2 * sin(xplus(1)) ^ 2 * sin(xplus(3)) * parDP.m1 * parDP.a1 * xplus(2) * xplus(6) - parDP.m2 * parDP.a2 * sin(xplus(3)) * xplus(4) * parDP.l1 * cos(xplus(1)) * xplus(2) * parDP.J1 - parDP.m2 * parDP.a2 * sin(xplus(3)) * xplus(4) * parDP.l1 * cos(xplus(1)) * xplus(2) * parDP.a1 ^ 2 * parDP.m1 + parDP.m2 * parDP.a2 * cos(xplus(3)) * xplus(4) * parDP.l1 * sin(xplus(1)) * xplus(2) * parDP.J1 + parDP.m2 * parDP.a2 * cos(xplus(3)) * xplus(4) * parDP.l1 * sin(xplus(1)) * xplus(2) * parDP.a1 ^ 2 * parDP.m1) / (parDP.J1 * parDP.m2 * parDP.a2 ^ 2 + parDP.J1 * parDP.J2 + parDP.a1 ^ 2 * parDP.m1 * parDP.m2 * parDP.a2 ^ 2 + parDP.a1 ^ 2 * parDP.m1 * parDP.J2 + parDP.m2 ^ 2 * parDP.l1 ^ 2 * parDP.a2 ^ 2 + parDP.m2 * parDP.l1 ^ 2 * parDP.J2 - parDP.m2 ^ 2 * parDP.l1 ^ 2 * parDP.a2 ^ 2 * cos(xplus(1)) ^ 2 * cos(xplus(3)) ^ 2 - 0.2e1 * parDP.m2 ^ 2 * parDP.l1 ^ 2 * parDP.a2 ^ 2 * cos(xplus(1)) * cos(xplus(3)) * sin(xplus(1)) * sin(xplus(3)) - parDP.m2 ^ 2 * parDP.l1 ^ 2 * parDP.a2 ^ 2 * sin(xplus(1)) ^ 2 * sin(xplus(3)) ^ 2) ^ 2 * (0.2e1 * parDP.m2 ^ 2 * parDP.l1 ^ 2 * parDP.a2 ^ 2 * cos(xplus(1)) ^ 2 * cos(xplus(3)) * sin(xplus(3)) + 0.2e1 * parDP.m2 ^ 2 * parDP.l1 ^ 2 * parDP.a2 ^ 2 * sin(xplus(1)) * sin(xplus(3)) ^ 2 * cos(xplus(1)) - 0.2e1 * parDP.m2 ^ 2 * parDP.l1 ^ 2 * parDP.a2 ^ 2 * cos(xplus(1)) * cos(xplus(3)) ^ 2 * sin(xplus(1)) - 0.2e1 * parDP.m2 ^ 2 * parDP.l1 ^ 2 * parDP.a2 ^ 2 * sin(xplus(1)) ^ 2 * cos(xplus(3)) * sin(xplus(3))) (-parDP.d2 * parDP.m2 * parDP.l1 ^ 2 - parDP.d2 * parDP.a1 ^ 2 * parDP.m1 - parDP.m2 ^ 2 * parDP.a2 * sin(xplus(3)) * parDP.l1 ^ 3 * cos(xplus(1)) * xplus(2) - parDP.m2 * parDP.l1 * parDP.a2 * cos(xplus(1)) * cos(xplus(3)) * parDP.d2 - parDP.m2 * parDP.l1 * parDP.a2 * sin(xplus(1)) * sin(xplus(3)) * parDP.d2 + parDP.m2 ^ 2 * parDP.a2 * cos(xplus(3)) * parDP.l1 ^ 3 * sin(xplus(1)) * xplus(2) + parDP.m2 * parDP.a2 * sin(xplus(3)) * xplus(6) * parDP.a1 ^ 2 * parDP.m1 + parDP.m2 * parDP.a2 * sin(xplus(3)) * xplus(6) * parDP.J1 + parDP.m2 ^ 2 * parDP.a2 * sin(xplus(3)) * xplus(6) * parDP.l1 ^ 2 - parDP.d2 * parDP.J1 - parDP.m2 ^ 2 * parDP.l1 ^ 2 * parDP.a2 ^ 2 * cos(xplus(1)) ^ 2 * cos(xplus(3)) * sin(xplus(3)) * xplus(2) - parDP.m2 ^ 2 * parDP.l1 ^ 2 * parDP.a2 ^ 2 * sin(xplus(1)) * sin(xplus(3)) ^ 2 * cos(xplus(1)) * xplus(2) + parDP.m2 ^ 2 * parDP.l1 ^ 2 * parDP.a2 ^ 2 * sin(xplus(1)) ^ 2 * sin(xplus(3)) * cos(xplus(3)) * xplus(2) + parDP.m2 ^ 2 * parDP.l1 ^ 2 * parDP.a2 ^ 2 * cos(xplus(1)) * cos(xplus(3)) ^ 2 * sin(xplus(1)) * xplus(2) - parDP.m2 * parDP.a2 * sin(xplus(3)) * parDP.l1 * cos(xplus(1)) * xplus(2) * parDP.J1 - parDP.m2 * parDP.a2 * sin(xplus(3)) * parDP.l1 * cos(xplus(1)) * xplus(2) * parDP.a1 ^ 2 * parDP.m1 + parDP.m2 * parDP.a2 * cos(xplus(3)) * parDP.l1 * sin(xplus(1)) * xplus(2) * parDP.J1 + parDP.m2 * parDP.a2 * cos(xplus(3)) * parDP.l1 * sin(xplus(1)) * xplus(2) * parDP.a1 ^ 2 * parDP.m1) / (parDP.J1 * parDP.m2 * parDP.a2 ^ 2 + parDP.J1 * parDP.J2 + parDP.a1 ^ 2 * parDP.m1 * parDP.m2 * parDP.a2 ^ 2 + parDP.a1 ^ 2 * parDP.m1 * parDP.J2 + parDP.m2 ^ 2 * parDP.l1 ^ 2 * parDP.a2 ^ 2 + parDP.m2 * parDP.l1 ^ 2 * parDP.J2 - parDP.m2 ^ 2 * parDP.l1 ^ 2 * parDP.a2 ^ 2 * cos(xplus(1)) ^ 2 * cos(xplus(3)) ^ 2 - 0.2e1 * parDP.m2 ^ 2 * parDP.l1 ^ 2 * parDP.a2 ^ 2 * cos(xplus(1)) * cos(xplus(3)) * sin(xplus(1)) * sin(xplus(3)) - parDP.m2 ^ 2 * parDP.l1 ^ 2 * parDP.a2 ^ 2 * sin(xplus(1)) ^ 2 * sin(xplus(3)) ^ 2) 0 (-parDP.m2 ^ 2 * parDP.l1 ^ 2 * parDP.a2 * sin(xplus(1)) ^ 2 * sin(xplus(3)) * xplus(2) + parDP.m2 * parDP.a2 * sin(xplus(3)) * xplus(4) * parDP.a1 ^ 2 * parDP.m1 + parDP.m2 * parDP.a2 * sin(xplus(3)) * xplus(4) * parDP.J1 + parDP.m2 ^ 2 * parDP.a2 * sin(xplus(3)) * xplus(4) * parDP.l1 ^ 2 - parDP.m2 * parDP.l1 * parDP.a2 * cos(xplus(1)) * cos(xplus(3)) * parDP.m1 * parDP.a1 * sin(xplus(1)) * xplus(2) - parDP.m2 ^ 2 * parDP.l1 ^ 2 * parDP.a2 * cos(xplus(1)) * cos(xplus(3)) * sin(xplus(1)) * xplus(2) - parDP.m2 * parDP.l1 * parDP.a2 * sin(xplus(1)) ^ 2 * sin(xplus(3)) * parDP.m1 * parDP.a1 * xplus(2)) / (parDP.J1 * parDP.m2 * parDP.a2 ^ 2 + parDP.J1 * parDP.J2 + parDP.a1 ^ 2 * parDP.m1 * parDP.m2 * parDP.a2 ^ 2 + parDP.a1 ^ 2 * parDP.m1 * parDP.J2 + parDP.m2 ^ 2 * parDP.l1 ^ 2 * parDP.a2 ^ 2 + parDP.m2 * parDP.l1 ^ 2 * parDP.J2 - parDP.m2 ^ 2 * parDP.l1 ^ 2 * parDP.a2 ^ 2 * cos(xplus(1)) ^ 2 * cos(xplus(3)) ^ 2 - 0.2e1 * parDP.m2 ^ 2 * parDP.l1 ^ 2 * parDP.a2 ^ 2 * cos(xplus(1)) * cos(xplus(3)) * sin(xplus(1)) * sin(xplus(3)) - parDP.m2 ^ 2 * parDP.l1 ^ 2 * parDP.a2 ^ 2 * sin(xplus(1)) ^ 2 * sin(xplus(3)) ^ 2)  ;
               0 0 0 0 0 1 ;
               0 0 0 0 0 0;];
end

== matlab function Doppelpendel_EKF/Modell/MATLAB Function ==
  data: u input; dx output; x input; parDP parameter
function dx = fcnDoppelpendel(u,x,parDP)
    %#codegen
    dx = Doppelpendel_NL_mfun(u,x,parDP);
end

== matlab function Doppelpendel_EKF/Vorsteuerung/Trajektorienplanung ==
  settings: updateMethod=DISCRETE  sampleTime=parLQR.Ta
  data: time input; deltax input; Te input; zz output; parFF parameter; uFF output; statesd output; start1 input; reset1 input; start2 input; start output; reset2 input; t output; start3 input; reset3 input
% Trajektorienplanung zum Versetzten des Doppelpendels
function [zz,uFF,statesd,start,t] = Trajektorienplanung(time,deltax,Te,parFF,start1,reset1,start2,reset2,start3,reset3)

persistent tstart
if isempty(tstart) tstart = double(0); end
persistent x0
if isempty(x0) x0 = double(0); end
persistent xT
if isempty(xT) xT = double(deltax); end


if reset1>0.5 || reset2>0.5 || reset3>0.5
    
    tstart = time;

end
%Zeit ab tstart
t = time - tstart;


if  start1>0.5 
    
    start = 1;
    
    if start2<0.5
        
        x0=0;
        xT=deltax; 
        
    else
        
        if start3<0.5
        
            x0=deltax;
            xT=-deltax; 
        
        else
    
            %Anfangs- und Endwert
            x0=-deltax;
            xT=deltax;
            
        end

    end
    
else
    
    start = 0;
    
end

% Folgendes hier bitte ausführen:
% 1.) Umrechnung auf Anfangs- und Endwert des Flachen Ausgangs
% 2.) Funktion Trajektorie() ergänzen
% 3.) Vorsteuerungsberechnung uFF ergänzen
% 4.) Sollzustandsverlauf statesd ergänzen

%Umrechnung auf Anfangs- und Endwert des Flachen Ausgangs
VV = inv(parFF.VVinv);
z0 = VV*x0;
zT = VV*xT;

z0 = z0(1);
zT = zT(1);

zz = Trajektorie(start,t,Te,z0,zT,parFF);
%zz=[z,zdot,z2dot,z3dot,z4dot,z5dot,z6dot];

%Vorsteuerung
uFF = parFF.aa' * zz';
%Sollzustandsverlauf
statesd =  parFF.VVinv * zz(1:6)';
end

%%%%%%%%%%%%%%%%%%%%%%%%%%%%%%%%%%%%%%%%%%%%%%%%%%%%%%%%%%%%%%%%%%%%%%%%%%    
function [zz] = Trajektorie(start,t,Te,z0,zT,parFF)
    
    if start<0.5

        z     = z0; 
        zdot  = 0; 
        z2dot = 0; 
        z3dot = 0; 
        z4dot = 0; 
        z5dot = 0; 
        z6dot = 0; 

    elseif start>0.5 && t<Te

        % Folgendes hier bitte ausführen:
        % 1.) Berechnung der Solltrajektorie
        beta_7 = parFF.beta7;
        beta_8 = parFF.beta8;
        beta_9 = parFF.beta9;
        beta_10 = parFF.beta10;
        beta_11 = parFF.beta11;
        beta_12 = parFF.beta12;
        beta_13 = parFF.beta13;
        Te = parFF.Te;

        zT_z0 = zT - z0;

        z = z0 + zT_z0 * (beta_7 * t ^ 7 / Te ^ 7 + beta_8 * t ^ 8 / Te ^ 8 + beta_9 * t ^ 9 / Te ^ 9 + beta_10 * t ^ 10 / Te ^ 10 + beta_11 * t ^ 11 / Te ^ 11 + beta_12 * t ^ 12 / Te ^ 12 + beta_13 * t ^ 13 / Te ^ 13);
        zdot = zT_z0 * (7 * beta_7 * t ^ 6 / Te ^ 7 + 8 * beta_8 * t ^ 7 / Te ^ 8 + 9 * beta_9 * t ^ 8 / Te ^ 9 + 10 * beta_10 * t ^ 9 / Te ^ 10 + 11 * beta_11 * t ^ 10 / Te ^ 11 + 12 * beta_12 * t ^ 11 / Te ^ 12 + 13 * beta_13 * t ^ 12 / Te ^ 13);
        z2dot = zT_z0 * (42 * beta_7 * t ^ 5 / Te ^ 7 + 56 * beta_8 * t ^ 6 / Te ^ 8 + 72 * beta_9 * t ^ 7 / Te ^ 9 + 90 * beta_10 * t ^ 8 / Te ^ 10 + 110 * beta_11 * t ^ 9 / Te ^ 11 + 132 * beta_12 * t ^ 10 / Te ^ 12 + 156 * beta_13 * t ^ 11 / Te ^ 13);
        z3dot = zT_z0 * (210 * beta_7 * t ^ 4 / Te ^ 7 + 336 * beta_8 * t ^ 5 / Te ^ 8 + 504 * beta_9 * t ^ 6 / Te ^ 9 + 720 * beta_10 * t ^ 7 / Te ^ 10 + 990 * beta_11 * t ^ 8 / Te ^ 11 + 1320 * beta_12 * t ^ 9 / Te ^ 12 + 1716 * beta_13 * t ^ 10 / Te ^ 13);
        z4dot = zT_z0 * (840 * beta_7 * t ^ 3 / Te ^ 7 + 1680 * beta_8 * t ^ 4 / Te ^ 8 + 3024 * beta_9 * t ^ 5 / Te ^ 9 + 5040 * beta_10 * t ^ 6 / Te ^ 10 + 7920 * beta_11 * t ^ 7 / Te ^ 11 + 11880 * beta_12 * t ^ 8 / Te ^ 12 + 17160 * beta_13 * t ^ 9 / Te ^ 13);
        z5dot = zT_z0 * (2520 * beta_7 * t ^ 2 / Te ^ 7 + 6720 * beta_8 * t ^ 3 / Te ^ 8 + 15120 * beta_9 * t ^ 4 / Te ^ 9 + 30240 * beta_10 * t ^ 5 / Te ^ 10 + 55440 * beta_11 * t ^ 6 / Te ^ 11 + 95040 * beta_12 * t ^ 7 / Te ^ 12 + 154440 * beta_13 * t ^ 8 / Te ^ 13);
        z6dot = zT_z0 * (5040 * beta_7 * t / Te ^ 7 + 20160 * beta_8 * t ^ 2 / Te ^ 8 + 60480 * beta_9 * t ^ 3 / Te ^ 9 + 151200 * beta_10 * t ^ 4 / Te ^ 10 + 332640 * beta_11 * t ^ 5 / Te ^ 11 + 665280 * beta_12 * t ^ 6 / Te ^ 12 + 1235520 * beta_13 * t ^ 7 / Te ^ 13);

        
    else

        z     = zT; 
        zdot  = 0; 
        z2dot = 0; 
        z3dot = 0; 
        z4dot = 0; 
        z5dot = 0; 
        z6dot = 0; 

    end

    zz=[z,zdot,z2dot,z3dot,z4dot,z5dot,z6dot];

end
